simulink model "adaptive_path_planning"  (R2026a)
settings: Solver=FixedStepDiscrete  StopTime=20  FixedStep=0.02
settings Model: Creator=itzke  LastModifiedBy=itzke

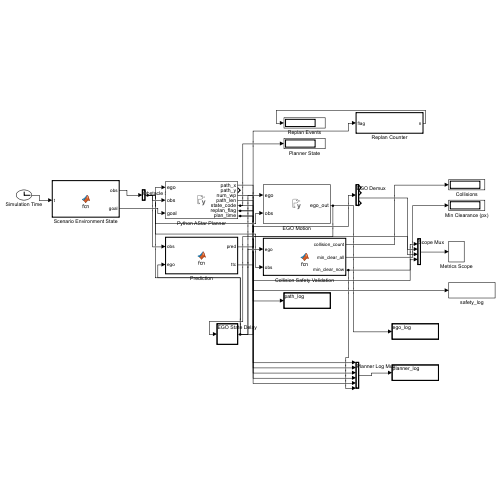
[thumbnail: Simulink's stored preview of the top-level diagram]
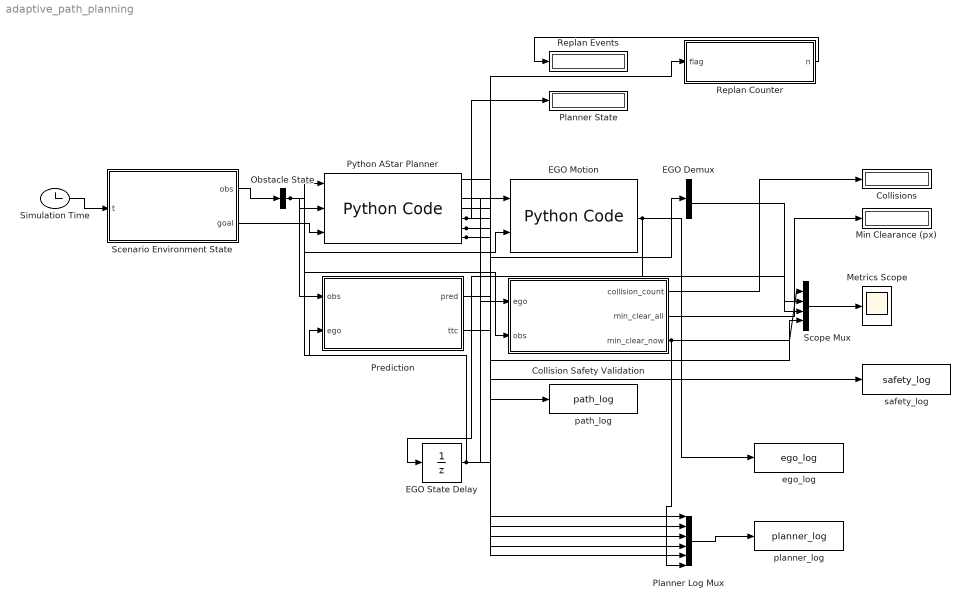
== system adaptive_path_planning ==
  Collision Safety Validation : MATLAB Function  TreatAsAtomicUnit=on
  Collisions : Display
  EGO Demux : Demux
  EGO Motion : PythonCode  InitializeConditionsCode=|  OutputCode=|  SampleTime=0.02
      InitializeConditionsCode=|
      | import sys, importlib
      | p = r"U:\\SIH-16-9-26-2-"
      | if p not in sys.path:
      |     sys.path.insert(0, p)
      | mb = importlib.import_module("matlab_bridge")
      | mb.initialize_planner()
      OutputCode=|
      | import numpy as np
      | mb.update_obstacles([[float(r[0]), float(r[1]), float(r[2]), float(r[3]), float(r[4])] for r in np.atleast_2d(obs) if r[0] > 0])
      | e = mb.ego_step(float(ego[0]), float(ego[1]), float(ego[2]), float(ego[3]), 0.02)
      | ego_out = np.array([e["x"], e["y"], e["v"], e["heading"]], dtype=float)
  EGO State Delay : UnitDelay  InitialCondition=[300;400;0;0]  SampleTime=0.02
  Metrics Scope : Scope
  Min Clearance (px) : Display
  Obstacle State : Mux  Inputs=1
  Planner Log Mux : Mux  Inputs=6
  Planner State : Display
  Prediction : MATLAB Function  TreatAsAtomicUnit=on
  Python AStar Planner : PythonCode  InitializeConditionsCode=|  OutputCode=|  SampleTime=0.2
      InitializeConditionsCode=|
      | import sys, importlib
      | p = r"U:\\SIH-16-9-26-2-"
      | if p not in sys.path:
      |     sys.path.insert(0, p)
      | mb = importlib.import_module("matlab_bridge")
      | mb.initialize_planner()
      OutputCode=|
      | import numpy as np
      | gx, gy = float(goal[0]), float(goal[1])
      | if mb._SESSION.goal != (gx, gy):
      |     mb.set_goal(gx, gy)
      | mb.update_obstacles([[float(r[0]), float(r[1]), float(r[2]), float(r[3]), float(r[4])] for r in np.atleast_2d(obs) if r[0] > 0])
      | r = mb.plan_path(float(ego[0]), float(ego[1]), float(ego[3]))
      | n = int(r["num_waypoints"]); m = min(n, 60)
      | px = np.full(60, np.nan); py = np.full(60, np.nan)
      | if m > 0:
      |     px[:m] = np.asarray(r["path_x"][:m], dtype=float)
      |     py[:m] = np.asarray(r["path_y"][:m], dtype=float)
      | path_x = px; path_y = py
      | num_wp = float(n); path_len = float(r["path_length_m"])
      | state_code = float(r["planner_state_code"])
      | replan_flag = 1.0 if r["replanned_this_call"] else 0.0
      | plan_time = 1000.0 * float(r["planning_time"])
  Replan Counter : MATLAB Function  TreatAsAtomicUnit=on
  Replan Events : Display
  Scenario Environment State : MATLAB Function  TreatAsAtomicUnit=on
  Scope Mux : Mux
  Simulation Time : Clock
  ego_log : ToWorkspace  VariableName=ego_log  SampleTime=-1
  path_log : ToWorkspace  VariableName=path_log  SampleTime=-1
  planner_log : ToWorkspace  VariableName=planner_log  SampleTime=-1
  safety_log : ToWorkspace  VariableName=safety_log  SampleTime=-1
  wires:
  Simulation Time/1 -> Scenario Environment State/1(t)
  Scenario Environment State/1(obs) -> Obstacle State/1
  Obstacle State/1 -> Prediction/1(obs), Python AStar Planner/2, EGO Motion/2, Collision Safety Validation/2(obs)
  Scenario Environment State/2(goal) -> Python AStar Planner/3
  EGO State Delay/1 -> Python AStar Planner/1, EGO Motion/1, Prediction/2(ego), Collision Safety Validation/1(ego), EGO Demux/1
  EGO Motion/1 -> EGO State Delay/1, ego_log/1
  Prediction/1(pred) -> safety_log/1
  Collision Safety Validation/1(collision_count) -> Collisions/1
  Collision Safety Validation/2(min_clear_all) -> Min Clearance (px)/1
  Collision Safety Validation/3(min_clear_now) -> Scope Mux/1, Planner Log Mux/6
  Python AStar Planner/5 -> Planner State/1, Planner Log Mux/3
  Python AStar Planner/6 -> Replan Counter/1(flag), Planner Log Mux/4
  Replan Counter/1(n) -> Replan Events/1
  Python AStar Planner/7 -> Scope Mux/2, Planner Log Mux/5
  Python AStar Planner/1 -> path_log/1
  Scope Mux/1 -> Metrics Scope/1
  EGO Demux/3 -> Scope Mux/3
  Prediction/2(ttc) -> Scope Mux/4
  Python AStar Planner/3 -> Planner Log Mux/1
  Python AStar Planner/4 -> Planner Log Mux/2
  Planner Log Mux/1 -> planner_log/1

== matlab function adaptive_path_planning/Prediction ==
  data: obs input; pred output; ego input; ttc output
function [pred, ttc] = fcn(obs, ego)                             
                                                                % Constant-velocity short-horizon prediction + time-to-collision.
                                                                H = 1.5;                                                         
                                                                pred = obs;                                                      
                                                                for i = 1:8                                                      
                                                                    if obs(i,1) > 0                                              
                                                                        pred(i,2) = obs(i,2) + obs(i,4)*cos(obs(i,5))*H;         
                                                                        pred(i,3) = obs(i,3) + obs(i,4)*sin(obs(i,5))*H;         
                                                                    end                                                          
                                                                end                                                              
                                                                ttc = inf;                                                       
                                                                fx = cos(ego(4)); fy = sin(ego(4));                              
                                                                for i = 1:8                                                      
                                                                    if obs(i,1) <= 0, continue; end                              
                                                                    rx = obs(i,2)-ego(1); ry = obs(i,3)-ego(2);                  
                                                                    along = rx*fx + ry*fy;                                       
                                                                    if along < 0, continue; end                                  
                                                                    ovx = obs(i,4)*cos(obs(i,5)); ovy = obs(i,4)*sin(obs(i,5));  
                                                                    closing = (ego(3)-ovx)*fx + (0-ovy)*fy;                      
                                                                    if closing > 1                                               
                                                                        ttc = min(ttc, along/closing);                           
                                                                    end                                                          
                                                                end

== matlab function adaptive_path_planning/Scenario Environment State ==
  data: t input; obs output; goal output
function [obs, goal] = fcn(t)                                                 
                                                                             % Indian-road validation scenario. Obstacle matrix rows:                      
                                                                             % [type_code, x(px), y(px), speed(px/s), heading(rad)]                        
                                                                             % codes: 1 car  2 truck  3 bus  4 auto_rickshaw  5 two_wheeler                
                                                                             %        6 bicycle  7 pedestrian  8 pushcart  9 animal  10 pothole            
                                                                             obs = zeros(8,5);                                                             
                                                                             obs(1,:) = [5, 700, 340, 0, 0];        % stopped two-wheeler (static blockage)
                                                                             obs(2,:) = [1, 1500 + 35*t, 420, 35, 0];  % moving car, same lane             
                                                                             obs(3,:) = [7, 1800, 330 + 10*t, 10, pi/2]; % pedestrian crossing             
                                                                             goal = [2500; 400];

== matlab function adaptive_path_planning/Collision Safety Validation ==
  data: ego input; collision_count output; obs input; min_clear_all output; min_clear_now output
function [collision_count, min_clear_all, min_clear_now] = fcn(ego, obs)  
                                                                         % Independent MATLAB-side safety validation (matches bridge radii).       
                                                                         persistent cc mc                                                          
                                                                         if isempty(cc), cc = 0; mc = inf; end                                     
                                                                         r = [19.8 30.8 34.1 15.4 11 11 3.85 12.1 13.2 16.5];                      
                                                                         mn = inf;                                                                 
                                                                         for i = 1:8                                                               
                                                                             if obs(i,1) <= 0, continue; end                                       
                                                                             d = hypot(ego(1)-obs(i,2), ego(2)-obs(i,3)) - 23 - r(int32(obs(i,1)));
                                                                             mn = min(mn, d);                                                      
                                                                         end                                                                       
                                                                         if mn < 0, cc = cc + 1; end                                               
                                                                         if mn < mc, mc = mn; end                                                  
                                                                         collision_count = cc; min_clear_all = mc; min_clear_now = mn;

== matlab function adaptive_path_planning/Replan Counter ==
  data: flag input; n output
function n = fcn(flag)                         
                                              persistent cnt prev                            
                                              if isempty(cnt), cnt = 0; prev = 0; end        
                                              if flag > 0.5 && prev < 0.5, cnt = cnt + 1; end
                                              prev = flag; n = cnt;
